simulink model "ED2_sim"  (R2013b)
settings: Solver=ode45  StartTime=0.0  StopTime=10  RelTol=1e-3
values from neighbouring files (symbols this model uses):
  A = [0 1 0 0 0 ... (first row only)    [vars_ed2.m]
  B = [0 0 ... (first row only)    [vars_ed2.m]
  C = [ 1 0 0 0 0 ... (first row only)    [vars_ed2.m]
  Ki = K(:,n+1:n+p)    [vars_ed2.m]
  Kp = K(:,1:n)    [vars_ed2.m]
settings Model: Creator=2022-0681  LastModifiedBy=2022-0681

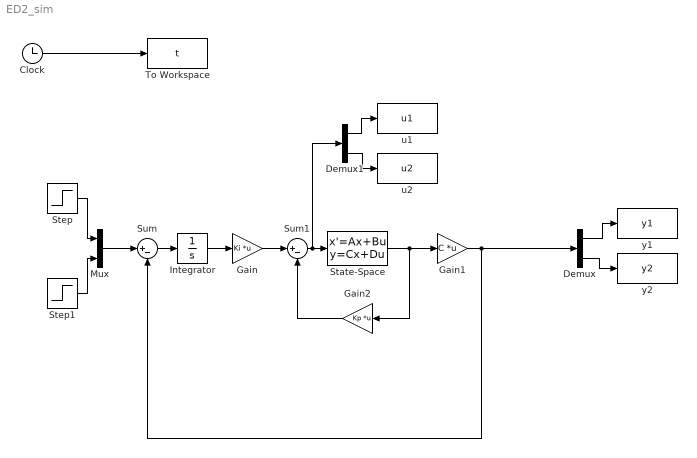
== system ED2_sim ==
  Clock : Clock
  Demux : Demux  Outputs=2
  Demux1 : Demux  Outputs=2
  Gain : Gain  Gain=Ki  Multiplication=Matrix(K*u) (u vector)
  Gain1 : Gain  Gain=C  Multiplication=Matrix(K*u) (u vector)
  Gain2 : Gain  Gain=Kp  Multiplication=Matrix(K*u) (u vector)
  Integrator : Integrator
  Mux : Mux  Inputs=2
  State-Space : StateSpace  A=A  B=B  C=eye(3)  D=zeros(3,2)  X0=0
  Step : Step  SampleTime=0
  Step1 : Step  Time=5  SampleTime=0
  Sum : Sum  Inputs=|+-
  Sum1 : Sum  Inputs=|+-
  To Workspace : ToWorkspace  VariableName=t  SampleTime=-1
  u1 : ToWorkspace  VariableName=u1  SampleTime=-1
  u2 : ToWorkspace  VariableName=u2  SampleTime=-1
  y1 : ToWorkspace  VariableName=y1  SampleTime=-1
  y2 : ToWorkspace  VariableName=y2  SampleTime=-1
  wires:
  Step/1 -> Mux/1
  Step1/1 -> Mux/2
  Mux/1 -> Sum/1
  State-Space/1 -> Gain2/1, Gain1/1
  Demux/1 -> y1/1
  Demux/2 -> y2/1
  Sum/1 -> Integrator/1
  Gain/1 -> Sum1/1
  Integrator/1 -> Gain/1
  Sum1/1 -> Demux1/1, State-Space/1
  Gain1/1 -> Sum/2, Demux/1
  Demux1/1 -> u1/1
  Demux1/2 -> u2/1
  Gain2/1 -> Sum1/2
  Clock/1 -> To Workspace/1
